simulink model "suspensionsytem"  (R2020b)
settings: Solver=VariableStepAuto  StartTime=0.0  StopTime=10.0  RelTol=1e-3
model workspace (MAT data in the model file):
  b = 50
  k1 = 50
  k2 = 20
  m1 = 0.01
  m2 = 0.001
settings Model: Creator=abhin  LastModifiedBy=abhin

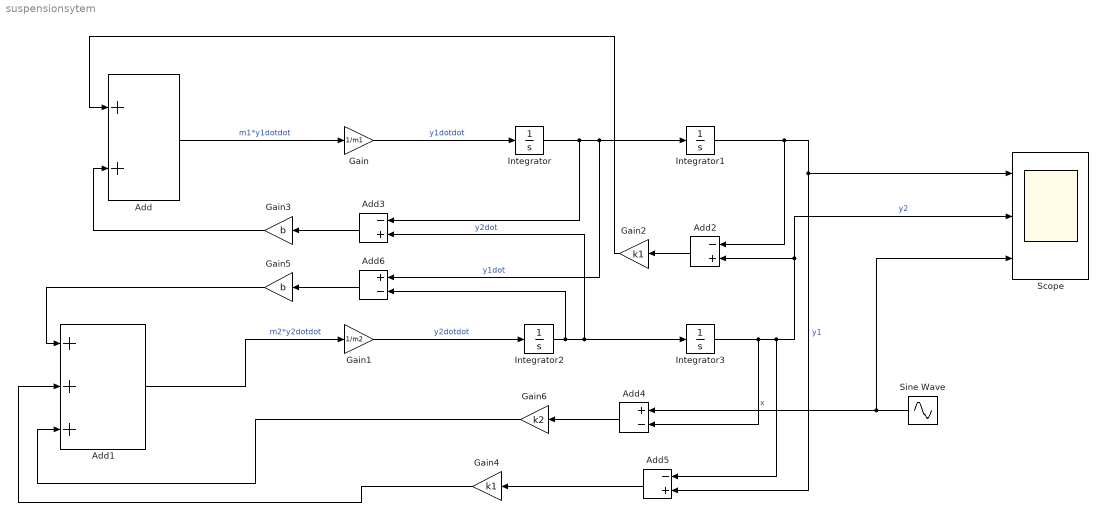
== system suspensionsytem ==
  Add : Sum
  Add1 : Sum  Inputs=+++
  Add2 : Sum  Inputs=-+
  Add3 : Sum  Inputs=-+
  Add4 : Sum  Inputs=+-
  Add5 : Sum  Inputs=-+
  Add6 : Sum  Inputs=+-
  Gain : Gain  Gain=1/m1
  Gain1 : Gain  Gain=1/m2
  Gain2 : Gain  Gain=k1
  Gain3 : Gain  Gain=b
  Gain4 : Gain  Gain=k1
  Gain5 : Gain  Gain=b
  Gain6 : Gain  Gain=k2
  Integrator{,1..3} (4 alike) : Integrator
  Scope : Scope  NumInputPorts=3
  Sine Wave : Sin  Amplitude=5  Frequency=2*pi*10  SampleTime=0
  wires:
  Add/1 -> Gain/1  "m1*y1dotdot"
  Gain/1 -> Integrator/1  "y1dotdot"
  Integrator/1 -> Add3/1, Add6/1, Integrator1/1  "y1dot"
  Integrator1/1 -> Add2/1, Add5/2, Scope/1  "y1"
  Add1/1 -> Gain1/1  "m2*y2dotdot"
  Gain1/1 -> Integrator2/1  "y2dotdot"
  Integrator2/1 -> Add6/2, Integrator3/1, Add3/2  "y2dot"
  Integrator3/1 -> Add4/2, Add5/1, Add2/2, Scope/2  "y2"
  Sine Wave/1 -> Scope/3, Add4/1  "x"
  Add4/1 -> Gain6/1
  Gain6/1 -> Add1/3
  Add2/1 -> Gain2/1
  Gain2/1 -> Add/1
  Add3/1 -> Gain3/1
  Gain3/1 -> Add/2
  Add5/1 -> Gain4/1
  Gain4/1 -> Add1/2
  Add6/1 -> Gain5/1
  Gain5/1 -> Add1/1
